simulink model "CLRC_filter_reg"  (R2024a)
settings: Solver=ode1  StartTime=0.0  StopTime=25  FixedStep=Ts  MaxStep=0.005  RelTol=1e-5
model workspace (MAT data in the model file):
  SL_ROS_VariableLengthArrays_MaxSizes.CommonInfo.ArrayTruncateAction = 'EmitWarning'
  SL_ROS_VariableLengthArrays_MaxSizes.MsgTypeMap = containers.Map
  SL_ROS_VariableLengthArrays_MaxSizes.MsgTypeMap.serialization.keys = {'gazebo_msgs/ApplyJointEffortRequest', 'sensor_msgs/JointState'}
  SL_ROS_VariableLengthArrays_MaxSizes.MsgTypeMap.serialization.values{1}.PropertyName = 'JointName'
  SL_ROS_VariableLengthArrays_MaxSizes.MsgTypeMap.serialization.values{1}.DataType = 'uint8'
  SL_ROS_VariableLengthArrays_MaxSizes.MsgTypeMap.serialization.values{1}.MaxLength = 12
  SL_ROS_VariableLengthArrays_MaxSizes.MsgTypeMap.serialization.values{2}(1).PropertyName = 'Effort'
  SL_ROS_VariableLengthArrays_MaxSizes.MsgTypeMap.serialization.values{2}(1).DataType = 'double'
  SL_ROS_VariableLengthArrays_MaxSizes.MsgTypeMap.serialization.values{2}(1).MaxLength = 128
  SL_ROS_VariableLengthArrays_MaxSizes.MsgTypeMap.serialization.values{2}(2).PropertyName = 'Name'
  SL_ROS_VariableLengthArrays_MaxSizes.MsgTypeMap.serialization.values{2}(2).DataType = 'std_msgs/String'
  SL_ROS_VariableLengthArrays_MaxSizes.MsgTypeMap.serialization.values{2}(2).MaxLength = 16
  SL_ROS_VariableLengthArrays_MaxSizes.MsgTypeMap.serialization.values{2}(3).PropertyName = 'Position'
  SL_ROS_VariableLengthArrays_MaxSizes.MsgTypeMap.serialization.values{2}(3).DataType = 'double'
  SL_ROS_VariableLengthArrays_MaxSizes.MsgTypeMap.serialization.values{2}(3).MaxLength = 7
  SL_ROS_VariableLengthArrays_MaxSizes.MsgTypeMap.serialization.values{2}(4).PropertyName = 'Velocity'
  SL_ROS_VariableLengthArrays_MaxSizes.MsgTypeMap.serialization.values{2}(4).DataType = 'double'
  SL_ROS_VariableLengthArrays_MaxSizes.MsgTypeMap.serialization.values{2}(4).MaxLength = 7
  SL_ROS_VariableLengthArrays_MaxSizes.MsgTypeMap.serialization.uniformity = 0
  SL_ROS_VariableLengthArrays_MaxSizes.MsgTypeMap.serialization.keyType = 'char'
  SL_ROS_VariableLengthArrays_MaxSizes.MsgTypeMap.serialization.valueType = 'any'
values from neighbouring files (symbols this model uses):
  alpha = 15    [Panda_run.m]
  alpha2 = 10    [Panda_run.m]
  dyn_par = opt_par()    [Panda_run.m]
  fricpar = FrictionPar()    [Panda_run.m]
  GammaW = 0.4*eye(N)    [Panda_run.m]
  invP = inv(P*P')*P    [Panda_run.m]
  kapa1 = 1    [Panda_run.m]
  kapa2 = 0    [Panda_run.m]
  Kc = diag([10,10,10,10,4,4,2.5])    [Panda_run.m]
  Lambda = 3*eye(7)    [Panda_run.m]
  P0 = 0.04    [Panda_run.m]
  P1 = 1    [Panda_run.m]
  q0 = [0, -0.60, 0, -2.25, 0, 1.5, 0.8]'    [Panda_run.m]
  robot_par = [basepar;fricpar]    [Panda_run.m]
  SD = 0.0    (= 0)    [Panda_run.m]
  taud = 25    [Panda_run.m]
  Ts = 0.0005    [Panda_run.m]
  vari = SD^2    [DDF_Test_main.m]    (also in Panda_run.m = 0; RegComp_main.m)
libraries: matrix_library x3
settings Model: SimulationMode=accelerator  Creator=STT  LastModifiedBy=SYSU-RCLLab-G
settings OptimizationCC: DefaultParameterBehavior=Inlined  EnhancedBackFolding=on  PassReuseOutputArgsAs=Individual arguments  ZeroExternalMemoryAtStartup=off  ZeroInternalMemoryAtStartup=off  MaxStackSize=64  AccelVerboseBuild=on  OptimizeBlockOrder=speed  DifferentSizesBufferReuse=on  OptimizationCustomize=off  EfficientTunableParamExpr=on
settings DebuggingCC: ArtificialAlgebraicLoopMsg=error  ParameterTunabilityLossMsg=error  UnconnectedInputMsg=warning  UnconnectedOutputMsg=warning  UnconnectedLineMsg=warning
settings ModelReferenceCC: EnableRefExpFcnMdlSchedulingChecks=on
settings SFSimCC: MATLABDynamicMemAlloc=off
settings RTWCC: Description=Embedded Coder  SystemTargetFile=ert.tlc  TemplateMakefile=ert_default_tmf  Toolchain=Catkin  GPUComputeCapability=3.5  DLArmComputeVersion=19.05
settings CodeAppCC: ForceParamTrailComments=on  IgnoreCustomStorageClasses=off  OperatorAnnotations=on  SimulinkDataObjDesc=on  SFDataObjDesc=on  InsertBlockDesc=on
settings ERTTargetCC: SupportContinuousTime=on  SupportVariableSizeSignals=on  ExtMode=on  ExtModeMexArgs='192.168.175.128' 0 17725  ERTCustomFileTemplate=example_file_process.tlc

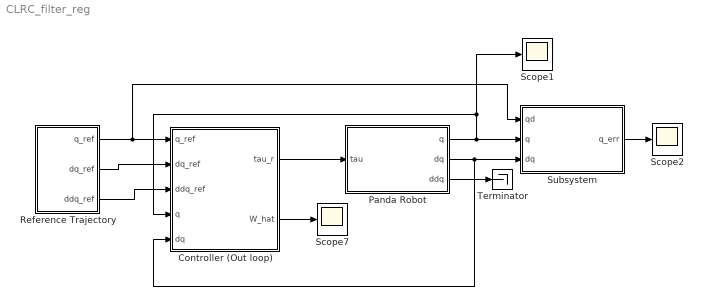
== system CLRC_filter_reg ==
  Controller (Out loop) : Subsystem  SystemSampleTime=1e-3
  Panda Robot : Subsystem
  Reference Trajectory : Subsystem
  Scope1 : Scope
  Scope2 : Scope
  Scope7 : Scope
  Subsystem : Subsystem
  Terminator : Terminator
  wires:
  Controller (Out loop)/2(W_hat) -> Scope7/1
  Controller (Out loop)/1(tau_r) -> Panda Robot/1(tau)
  Reference Trajectory/1(q_ref) -> Subsystem/1(qd), Controller (Out loop)/1(q_ref)
  Reference Trajectory/2(dq_ref) -> Controller (Out loop)/2(dq_ref)
  Reference Trajectory/3(ddq_ref) -> Controller (Out loop)/3(ddq_ref)
  Panda Robot/2(dq) -> Subsystem/3(dq), Controller (Out loop)/5(dq)
  Subsystem/1(q_err) -> Scope2/1
  Panda Robot/1(q) -> Scope1/1, Controller (Out loop)/4(q), Subsystem/2(q)
  Panda Robot/3(ddq) -> Terminator/1

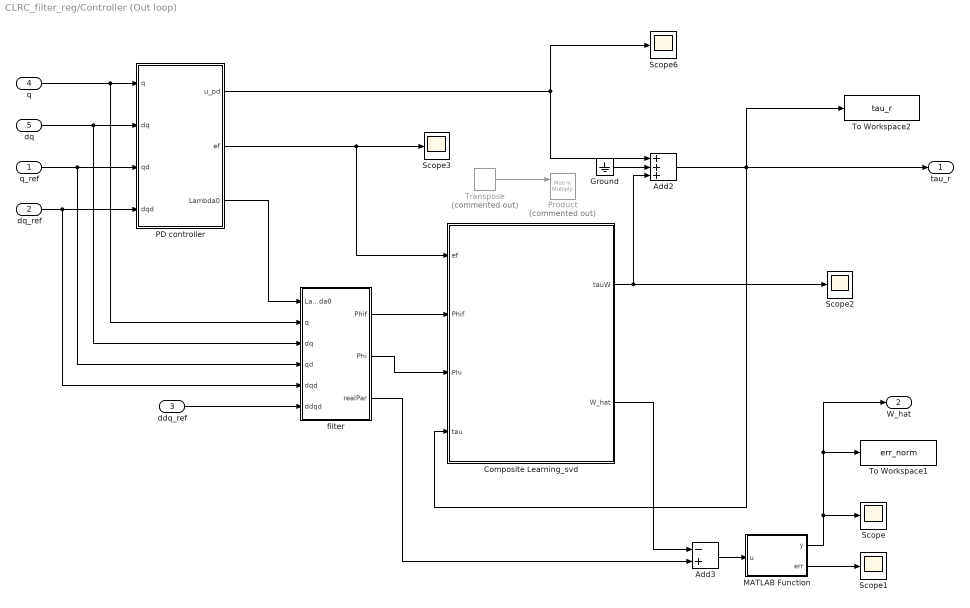
== system CLRC_filter_reg/Controller (Out loop) ==
  q_ref : Inport
  dq_ref : Inport  Port=2
  ddq_ref : Inport  Port=3
  q : Inport  Port=4
  dq : Inport  Port=5
  Add2 : Sum  Inputs=+++
  Add3 : Sum  Inputs=-+
  Composite Learning_svd : Subsystem
  Ground : Ground
  MATLAB Function : MATLAB Function  TreatAsAtomicUnit=on
  PD controller : Subsystem
  Product : Product  Commented=on  Multiplication=Matrix(*)
  Scope{,1..3,6} (5 alike) : Scope
  To Workspace1 : ToWorkspace  VariableName=err_norm  SaveFormat=Timeseries  SampleTime=-1
  To Workspace2 : ToWorkspace  VariableName=tau_r  SaveFormat=Timeseries  SampleTime=-1
  Transpose : matrix_library/Transpose  Commented=on
  filter : Subsystem
  tau_r : Outport
  W_hat : Outport  Port=2
  wires:
  q_ref/1 -> filter/4(qd), PD controller/3(qd)
  dq_ref/1 -> filter/5(dqd), PD controller/4(dqd)
  dq/1 -> filter/3(dq), PD controller/2(dq)
  ddq_ref/1 -> filter/6(ddqd)
  Add3/1 -> MATLAB Function/1(u)
  MATLAB Function/1(y) -> W_hat/1, To Workspace1/1, Scope/1
  filter/1(Phif) -> Composite Learning_svd/2(Phif)
  filter/2(Phi) -> Composite Learning_svd/3(Phi)
  MATLAB Function/2(err) -> Scope1/1
  filter/3(realPar) -> Add3/2
  Transpose/1 -> Product/1
  Composite Learning_svd/1(tauW) -> Add2/3, Scope2/1
  q/1 -> filter/2(q), PD controller/1(q)
  Composite Learning_svd/2(W_hat) -> Add3/1
  Add2/1 -> Composite Learning_svd/4(tau), tau_r/1, To Workspace2/1
  PD controller/3(Lambda0) -> filter/1(Lambda0)
  PD controller/2(ef) -> Scope3/1, Composite Learning_svd/1(ef)
  PD controller/1(u_pd) -> Add2/1, Scope6/1
  Ground/1 -> Add2/2

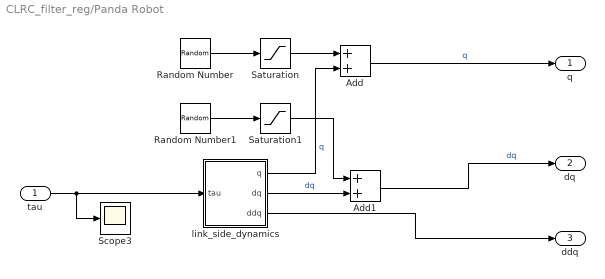
== system CLRC_filter_reg/Panda Robot ==
  tau : Inport
  Add : Sum
  Add1 : Sum
  Random Number : RandomNumber  Variance=vari  SampleTime=Ts
  Random Number1 : RandomNumber  Variance=vari  SampleTime=Ts
  Saturation : Saturate  UpperLimit=3*SD  LowerLimit=-3*SD
  Saturation1 : Saturate  UpperLimit=3*SD  LowerLimit=-3*SD
  Scope3 : Scope
  link_side_dynamics : Subsystem
  q : Outport
  dq : Outport  Port=2
  ddq : Outport  Port=3
  wires:
  link_side_dynamics/1(q) -> Add/2  "q"
  tau/1 -> link_side_dynamics/1(tau), Scope3/1
  Random Number/1 -> Saturation/1
  Saturation/1 -> Add/1
  Random Number1/1 -> Saturation1/1
  link_side_dynamics/2(dq) -> Add1/2  "dq"
  Add/1 -> q/1  "q"
  Add1/1 -> dq/1  "dq"
  Saturation1/1 -> Add1/1
  link_side_dynamics/3(ddq) -> ddq/1

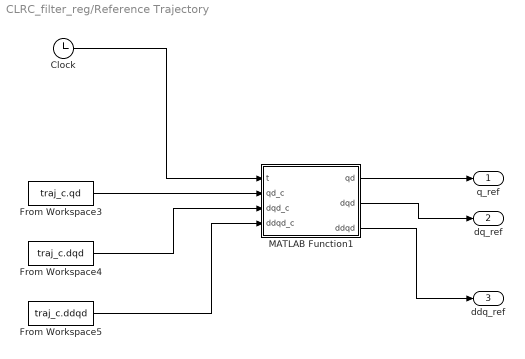
== system CLRC_filter_reg/Reference Trajectory ==
  Clock : Clock
  From Workspace3 : FromWorkspace  VariableName=traj_c.qd
  From Workspace4 : FromWorkspace  VariableName=traj_c.dqd
  From Workspace5 : FromWorkspace  VariableName=traj_c.ddqd
  MATLAB Function1 : MATLAB Function  TreatAsAtomicUnit=on
  q_ref : Outport
  dq_ref : Outport  Port=2
  ddq_ref : Outport  Port=3
  wires:
  Clock/1 -> MATLAB Function1/1(t)
  MATLAB Function1/1(qd) -> q_ref/1
  MATLAB Function1/2(dqd) -> dq_ref/1
  MATLAB Function1/3(ddqd) -> ddq_ref/1
  From Workspace3/1 -> MATLAB Function1/2(qd_c)
  From Workspace4/1 -> MATLAB Function1/3(dqd_c)
  From Workspace5/1 -> MATLAB Function1/4(ddqd_c)

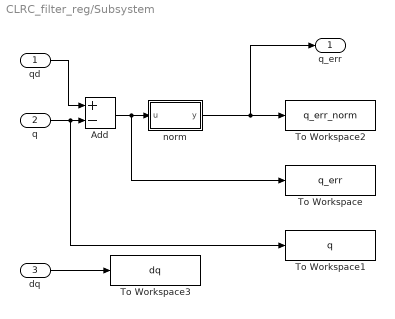
== system CLRC_filter_reg/Subsystem ==
  qd : Inport
  q : Inport  Port=2
  dq : Inport  Port=3
  Add : Sum  Inputs=+-
  To Workspace : ToWorkspace  VariableName=q_err  SaveFormat=Timeseries  SampleTime=-1
  To Workspace1 : ToWorkspace  VariableName=q  SaveFormat=Timeseries  SampleTime=-1
  To Workspace2 : ToWorkspace  VariableName=q_err_norm  SaveFormat=Timeseries  SampleTime=-1
  To Workspace3 : ToWorkspace  VariableName=dq  SaveFormat=Timeseries  SampleTime=-1
  norm : MATLAB Function  TreatAsAtomicUnit=on
  q_err : Outport
  wires:
  norm/1(y) -> q_err/1, To Workspace2/1
  q/1 -> To Workspace1/1, Add/2
  qd/1 -> Add/1
  Add/1 -> norm/1(u), To Workspace/1
  dq/1 -> To Workspace3/1

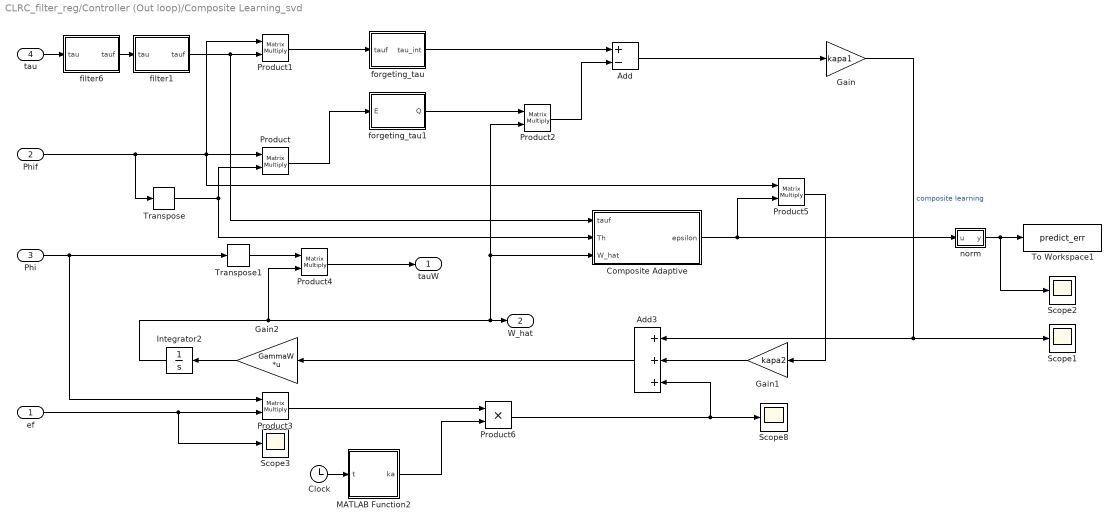
== system CLRC_filter_reg/Controller (Out loop)/Composite Learning_svd ==
  ef : Inport
  Phif : Inport  Port=2
  Phi : Inport  Port=3
  tau : Inport  Port=4
  Add : Sum  Inputs=+-
  Add3 : Sum  Inputs=+++
  Clock : Clock
  Composite Adaptive : Subsystem
  Gain : Gain  Gain=kapa1
  Gain1 : Gain  Gain=kapa2
  Gain2 : Gain  Gain=GammaW  Multiplication=Matrix(K*u)
  Integrator2 : Integrator  UpperSaturationLimit=10  LowerSaturationLimit=-1
  MATLAB Function2 : MATLAB Function  TreatAsAtomicUnit=on
  Product{,1..5} (6 alike) : Product  Multiplication=Matrix(*)
  Product6 : Product
  Scope{1..3,8} (4 alike) : Scope
  To Workspace1 : ToWorkspace  VariableName=predict_err  SaveFormat=Timeseries  SampleTime=-1
  Transpose : matrix_library/Transpose
  Transpose1 : matrix_library/Transpose
  filter1 : Subsystem
  filter6 : Subsystem
  forgeting_tau : Subsystem
  forgeting_tau1 : Subsystem
  norm : MATLAB Function  TreatAsAtomicUnit=on
  tauW : Outport
  W_hat : Outport  Port=2
  wires:
  Transpose/1 -> Composite Adaptive/2(Th), Product/2
  ef/1 -> Scope3/1, Product3/2
  Phi/1 -> Transpose1/1, Product3/1
  Transpose1/1 -> Product4/1
  Phif/1 -> Product1/1, Product5/1, Product/1, Transpose/1
  Gain2/1 -> Integrator2/1
  Add3/1 -> Gain2/1
  Composite Adaptive/1(epsilon) -> Product5/2, norm/1(u)
  Product4/1 -> tauW/1
  norm/1(y) -> Scope2/1, To Workspace1/1
  tau/1 -> filter6/1(tau)
  filter1/1(tauf) -> Composite Adaptive/1(tauf), Product1/2
  Product3/1 -> Product6/1
  Gain/1 -> Add3/1, Scope1/1  "composite learning"
  Integrator2/1 -> Product4/2, Product2/2, Composite Adaptive/3(W_hat), W_hat/1
  Product/1 -> forgeting_tau1/1(E)
  Product1/1 -> forgeting_tau/1(tauf)
  forgeting_tau1/1(Q) -> Product2/1
  forgeting_tau/1(tau_int) -> Add/1
  Product2/1 -> Add/2
  Add/1 -> Gain/1
  filter6/1(tauf) -> filter1/1(tau)
  Clock/1 -> MATLAB Function2/1(t)
  MATLAB Function2/1(ka) -> Product6/2
  Product5/1 -> Gain1/1
  Product6/1 -> Add3/3, Scope8/1
  Gain1/1 -> Add3/2

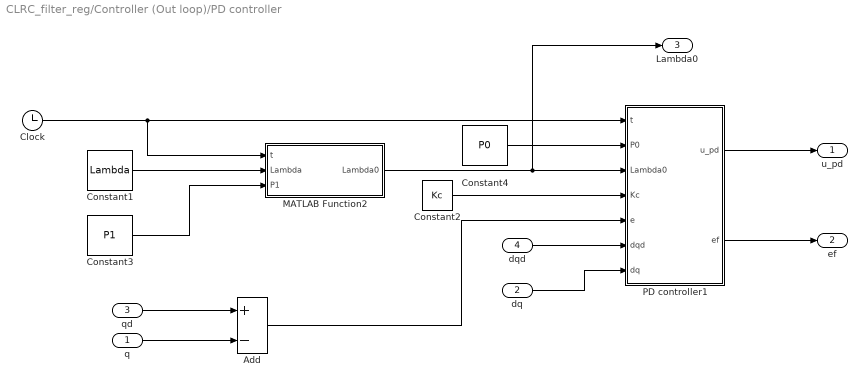
== system CLRC_filter_reg/Controller (Out loop)/PD controller ==
  q : Inport
  dq : Inport  Port=2
  qd : Inport  Port=3
  dqd : Inport  Port=4
  Add : Sum  Inputs=+-
  Clock : Clock
  Constant1 : Constant  Value=Lambda
  Constant2 : Constant  Value=Kc
  Constant3 : Constant  Value=P1
  Constant4 : Constant  Value=P0
  MATLAB Function2 : MATLAB Function  TreatAsAtomicUnit=on
  PD controller1 : MATLAB Function  TreatAsAtomicUnit=on
  u_pd : Outport
  ef : Outport  Port=2
  Lambda0 : Outport  Port=3
  wires:
  PD controller1/1(u_pd) -> u_pd/1
  Constant4/1 -> PD controller1/2(P0)
  Clock/1 -> MATLAB Function2/1(t), PD controller1/1(t)
  Add/1 -> PD controller1/5(e)
  MATLAB Function2/1(Lambda0) -> Lambda0/1, PD controller1/3(Lambda0)
  Constant1/1 -> MATLAB Function2/2(Lambda)
  Constant3/1 -> MATLAB Function2/3(P1)
  Constant2/1 -> PD controller1/4(Kc)
  PD controller1/2(ef) -> ef/1
  q/1 -> Add/2
  qd/1 -> Add/1
  dq/1 -> PD controller1/7(dq)
  dqd/1 -> PD controller1/6(dqd)

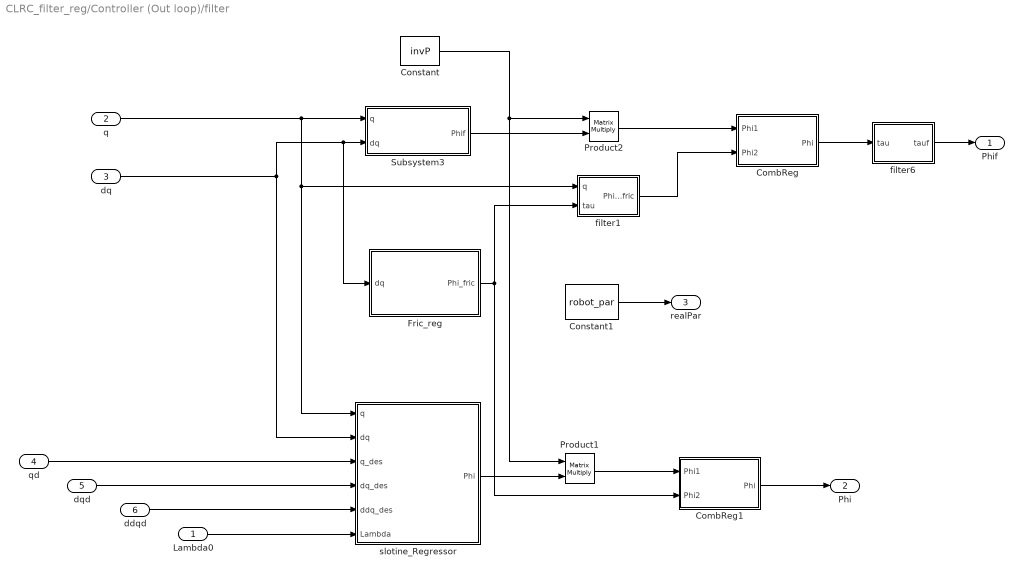
== system CLRC_filter_reg/Controller (Out loop)/filter ==
  Lambda0 : Inport
  q : Inport  Port=2
  dq : Inport  Port=3
  qd : Inport  Port=4
  dqd : Inport  Port=5
  ddqd : Inport  Port=6
  CombReg : MATLAB Function  TreatAsAtomicUnit=on
  CombReg1 : MATLAB Function  TreatAsAtomicUnit=on
  Constant : Constant  Value=invP
  Constant1 : Constant  Value=robot_par
  Fric_reg : MATLAB Function  TreatAsAtomicUnit=on
  Product1 : Product  Multiplication=Matrix(*)
  Product2 : Product  Multiplication=Matrix(*)
  Subsystem3 : Subsystem
  filter1 : Subsystem
  filter6 : Subsystem
  slotine_Regressor : MATLAB Function  TreatAsAtomicUnit=on
  Phif : Outport
  Phi : Outport  Port=2
  realPar : Outport  Port=3
  wires:
  qd/1 -> slotine_Regressor/3(q_des)
  dqd/1 -> slotine_Regressor/4(dq_des)
  ddqd/1 -> slotine_Regressor/5(ddq_des)
  Lambda0/1 -> slotine_Regressor/6(Lambda)
  q/1 -> filter1/1(q), slotine_Regressor/1(q), Subsystem3/1(q)
  dq/1 -> Fric_reg/1(dq), Subsystem3/2(dq), slotine_Regressor/2(dq)
  Constant1/1 -> realPar/1
  filter6/1(tauf) -> Phif/1
  Fric_reg/1(Phi_fric) -> filter1/2(tau), CombReg1/2(Phi2)
  filter1/1(Phif_fric) -> CombReg/2(Phi2)
  slotine_Regressor/1(Phi) -> Product1/2
  CombReg/1(Phi) -> filter6/1(tau)
  CombReg1/1(Phi) -> Phi/1
  Constant/1 -> Product2/1, Product1/1
  Product1/1 -> CombReg1/1(Phi1)
  Product2/1 -> CombReg/1(Phi1)
  Subsystem3/1(Phif) -> Product2/2

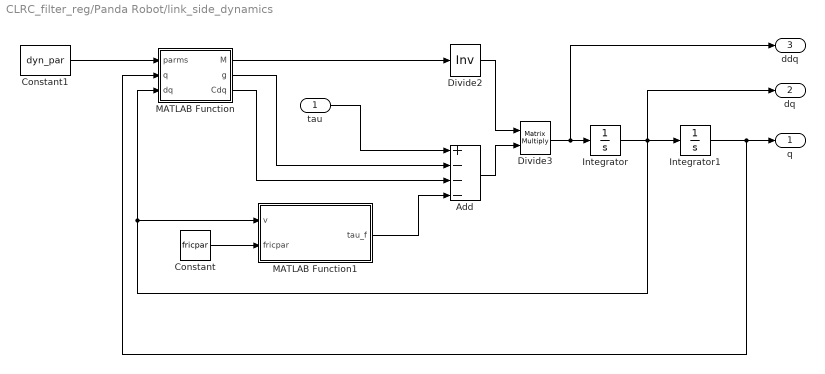
== system CLRC_filter_reg/Panda Robot/link_side_dynamics ==
  tau : Inport
  Add : Sum  Inputs=+---
  Constant : Constant  Value=fricpar
  Constant1 : Constant  Value=dyn_par
  Divide2 : Product  Inputs=/  Multiplication=Matrix(*)
  Divide3 : Product  Inputs=**  Multiplication=Matrix(*)
  Integrator : Integrator  InitialCondition=zeros(7,1)
  Integrator1 : Integrator  InitialCondition=q0
  MATLAB Function : MATLAB Function  TreatAsAtomicUnit=on
  MATLAB Function1 : MATLAB Function  TreatAsAtomicUnit=on
  q : Outport
  dq : Outport  Port=2
  ddq : Outport  Port=3
  wires:
  Divide3/1 -> Integrator/1, ddq/1
  tau/1 -> Add/1
  Integrator1/1 -> q/1, MATLAB Function/2(q)
  Constant/1 -> MATLAB Function1/2(fricpar)
  Add/1 -> Divide3/2
  Divide2/1 -> Divide3/1
  MATLAB Function1/1(tau_f) -> Add/4
  Integrator/1 -> MATLAB Function/3(dq), MATLAB Function1/1(v), Integrator1/1, dq/1
  MATLAB Function/1(M) -> Divide2/1
  MATLAB Function/3(Cdq) -> Add/3
  Constant1/1 -> MATLAB Function/1(parms)
  MATLAB Function/2(g) -> Add/2

== system CLRC_filter_reg/Controller (Out loop)/Composite Learning_svd/Composite Adaptive ==
  tauf : Inport
  Th : Inport  Port=2
  W_hat : Inport  Port=3
  Add1 : Sum  Inputs=+-
  Product6 : Product  Multiplication=Matrix(*)
  epsilon : Outport
  wires:
  Add1/1 -> epsilon/1
  Product6/1 -> Add1/2
  tauf/1 -> Add1/1
  Th/1 -> Product6/1
  W_hat/1 -> Product6/2

== system CLRC_filter_reg/Controller (Out loop)/Composite Learning_svd/filter1 ==
  tau : Inport
  Add : Sum  Inputs=+-
  Gain : Gain  Gain=alpha2
  Integrator : Integrator  UpperSaturationLimit=20  LowerSaturationLimit=-20
  tauf : Outport
  wires:
  tau/1 -> Add/1
  Add/1 -> Gain/1
  Gain/1 -> Integrator/1
  Integrator/1 -> Add/2, tauf/1

== system CLRC_filter_reg/Controller (Out loop)/Composite Learning_svd/filter6 ==
  tau : Inport
  Add : Sum  Inputs=+-
  Gain : Gain  Gain=alpha
  Integrator : Integrator  UpperSaturationLimit=20  LowerSaturationLimit=-20
  tauf : Outport
  wires:
  tau/1 -> Add/1
  Add/1 -> Gain/1
  Gain/1 -> Integrator/1
  Integrator/1 -> Add/2, tauf/1

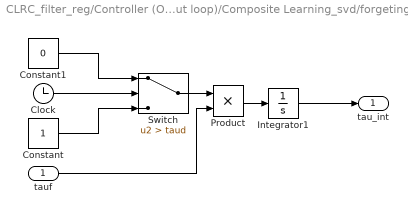
== system CLRC_filter_reg/Controller (Out loop)/Composite Learning_svd/forgeting_tau ==
  tauf : Inport
  Clock : Clock
  Constant : Constant
  Constant1 : Constant  Value=0
  Integrator1 : Integrator  UpperSaturationLimit=20  LowerSaturationLimit=-20
  Product : Product
  Switch : Switch  Criteria=u2 > Threshold  Threshold=taud  SaturateOnIntegerOverflow=off  InputSameDT=off
  tau_int : Outport
  wires:
  tauf/1 -> Product/2
  Clock/1 -> Switch/2
  Integrator1/1 -> tau_int/1
  Constant/1 -> Switch/3
  Constant1/1 -> Switch/1
  Switch/1 -> Product/1
  Product/1 -> Integrator1/1

== system CLRC_filter_reg/Controller (Out loop)/Composite Learning_svd/forgeting_tau1 ==
  E : Inport
  Clock : Clock
  Constant : Constant
  Constant1 : Constant  Value=0
  Integrator1 : Integrator  UpperSaturationLimit=20  LowerSaturationLimit=-20
  Product : Product
  Switch : Switch  Criteria=u2 > Threshold  Threshold=taud  SaturateOnIntegerOverflow=off  InputSameDT=off
  Q : Outport
  wires:
  E/1 -> Product/2
  Clock/1 -> Switch/2
  Integrator1/1 -> Q/1
  Constant/1 -> Switch/3
  Constant1/1 -> Switch/1
  Switch/1 -> Product/1
  Product/1 -> Integrator1/1

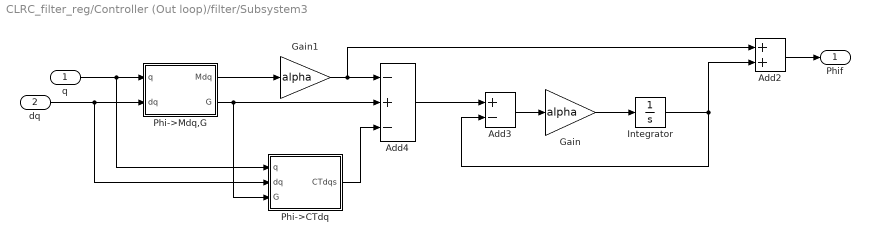
== system CLRC_filter_reg/Controller (Out loop)/filter/Subsystem3 ==
  q : Inport
  dq : Inport  Port=2
  Add2 : Sum
  Add3 : Sum  Inputs=+-
  Add4 : Sum  Inputs=-+-
  Gain : Gain  Gain=alpha
  Gain1 : Gain  Gain=alpha
  Integrator : Integrator  UpperSaturationLimit=20  LowerSaturationLimit=-20
  Phi->CTdq : MATLAB Function  TreatAsAtomicUnit=on
  Phi->Mdq,G : MATLAB Function  TreatAsAtomicUnit=on
  Phif : Outport
  wires:
  Add4/1 -> Add3/1
  Add2/1 -> Phif/1
  Add3/1 -> Gain/1
  Gain/1 -> Integrator/1
  q/1 -> Phi->CTdq/1(q), Phi->Mdq,G/1(q)
  dq/1 -> Phi->CTdq/2(dq), Phi->Mdq,G/2(dq)
  Phi->Mdq,G/1(Mdq) -> Gain1/1
  Gain1/1 -> Add2/1, Add4/1
  Integrator/1 -> Add2/2, Add3/2
  Phi->CTdq/1(CTdqs) -> Add4/3
  Phi->Mdq,G/2(G) -> Add4/2, Phi->CTdq/3(G)

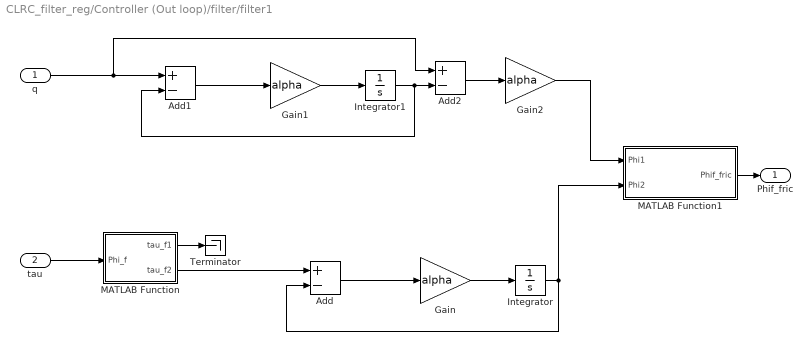
== system CLRC_filter_reg/Controller (Out loop)/filter/filter1 ==
  q : Inport
  tau : Inport  Port=2
  Add : Sum  Inputs=+-
  Add1 : Sum  Inputs=+-
  Add2 : Sum  Inputs=+-
  Gain : Gain  Gain=alpha
  Gain1 : Gain  Gain=alpha
  Gain2 : Gain  Gain=alpha
  Integrator : Integrator  UpperSaturationLimit=20  LowerSaturationLimit=-20
  Integrator1 : Integrator  InitialCondition=q0  UpperSaturationLimit=20  LowerSaturationLimit=-20
  MATLAB Function : MATLAB Function  TreatAsAtomicUnit=on
  MATLAB Function1 : MATLAB Function  TreatAsAtomicUnit=on
  Terminator : Terminator
  Phif_fric : Outport
  wires:
  Add/1 -> Gain/1
  Gain/1 -> Integrator/1
  Integrator/1 -> MATLAB Function1/2(Phi2), Add/2
  tau/1 -> MATLAB Function/1(Phi_f)
  MATLAB Function/2(tau_f2) -> Add/1
  Integrator1/1 -> Add1/2, Add2/2
  Gain1/1 -> Integrator1/1
  Add1/1 -> Gain1/1
  q/1 -> Add1/1, Add2/1
  Add2/1 -> Gain2/1
  MATLAB Function1/1(Phif_fric) -> Phif_fric/1
  Gain2/1 -> MATLAB Function1/1(Phi1)
  MATLAB Function/1(tau_f1) -> Terminator/1

== system CLRC_filter_reg/Controller (Out loop)/filter/filter6 ==
  tau : Inport
  Add : Sum  Inputs=+-
  Gain : Gain  Gain=alpha2
  Integrator : Integrator  UpperSaturationLimit=20  LowerSaturationLimit=-20
  tauf : Outport
  wires:
  tau/1 -> Add/1
  Add/1 -> Gain/1
  Gain/1 -> Integrator/1
  Integrator/1 -> Add/2, tauf/1

== matlab function CLRC_filter_reg/Controller (Out loop)/filter/CombReg1 ==
  data: Phi1 input; Phi output; Phi2 input
function Phi = fcn(Phi1,Phi2)

Phi = [Phi1;Phi2];

== matlab function CLRC_filter_reg/Controller (Out loop)/filter/filter1/MATLAB Function ==
  data: Phi_f input; tau_f1 output; tau_f2 output
function [tau_f1,tau_f2] = fcn(Phi_f)
tau_f1=Phi_f(1:7,:);
tau_f2 = Phi_f(8:end,:);

== matlab function CLRC_filter_reg/Controller (Out loop)/filter/filter1/MATLAB Function1 ==
  data: Phi1 input; Phif_fric output; Phi2 input
function Phif_fric = fcn(Phi1,Phi2)
Phif_fric=[diag(Phi1);Phi2];

== matlab function CLRC_filter_reg/Controller (Out loop)/Composite Learning_svd/MATLAB Function2 ==
  data: t input; ka output
function ka= fcn(t)


if t<40
    ka=1;
elseif t<100
    ka=1-0.5*(1+tanh((t-70)/5));
else
    ka=0;
end

== matlab function CLRC_filter_reg/Controller (Out loop)/PD controller/PD controller1 ==
  data: t input; P0 input; Lambda0 input; Kc input; e input; dqd input; u_pd output; dq input; ef output
function [u_pd,ef]= fcn(t,P0,Lambda0,Kc,e,dqd,dq)


%% Kc
% P0=0.02;
if t<40
    Kc0=Kc;
elseif t<100
    Kc0=Kc-0.5*(1+tanh((t-70)/5))*(1-P0)*Kc;
else
    Kc0=P0*Kc;
end
dqr=(dqd+Lambda0*e);

ef=dqr-dq;

u_pd = Kc0*ef;

== matlab function CLRC_filter_reg/Panda Robot/link_side_dynamics/MATLAB Function ==
  data: parms input; M output; q input; dq input; g output; Cdq output
function [M,g,Cdq] = fcn(parms,q,dq)

M= Mass(parms,q);

g=gravity(parms,q);

Cdq= CoriolisVector(parms,q,dq);

== matlab function CLRC_filter_reg/Controller (Out loop)/MATLAB Function ==
  data: u input; y output; err output
function [y,err]= fcn(u)

y = norm(u);
err=abs(u);

== matlab function CLRC_filter_reg/Controller (Out loop)/PD controller/MATLAB Function2 ==
  data: t input; Lambda0 output; Lambda input; P1 input
function Lambda0= fcn(t,Lambda,P1)


if t<40
    Lambda0=Lambda;
elseif t<100
    Lambda0=Lambda-0.5*(1+tanh((t-70)/5))*(1-P1)*Lambda;
else
    Lambda0=P1*Lambda;
end

== matlab function CLRC_filter_reg/Controller (Out loop)/filter/Subsystem3/Phi->Mdq,G ==
  data: q input; Mdq output; dq input; G output
function [Mdq,G] = fcn(q,dq)


vec0=zeros(7,1);


% G=Base_Regressor_Panda_43(q,vec0,vec0);
% Mdq=Base_Regressor_Panda_43(q,vec0,dq)-G;
G=Regressor_Panda_full(q,vec0,vec0);

Mdq=Regressor_Panda_full(q,vec0,dq)-G;

== matlab function CLRC_filter_reg/Subsystem/norm ==
  data: u input; y output
function y = fcn(u)

y = norm(u);

== matlab function CLRC_filter_reg/Panda Robot/link_side_dynamics/MATLAB Function1 ==
  data: v input; tau_f output; fricpar input
function tau_f = signFriction(v,fricpar)
 % f_v =[0.0665, 0.1987, 0.0399, 0.2257,  0.1023, -0.0132, 0.0638]';
 % f_c =[0.245, 0.1523, 0.1827, 0.3591, 0.2669, 0.1658, 0.2109 ]';
 % f_o =[-0.1073,-0.1566,-0.0686,-0.2522,0.0045,0.0910,-0.0127]';
 % tau_f = f_v.*v+f_c.*tanh(300*v)+f_o;


 tau_f = Regressor_fric(v)'*fricpar;

== matlab function CLRC_filter_reg/Controller (Out loop)/filter/Fric_reg ==
  data: dq input; Phi_fric output
function Phi_fric = fcn(dq)

Phi_fric = Regressor_fric(dq);

== matlab function CLRC_filter_reg/Controller (Out loop)/filter/slotine_Regressor ==
  data: q input; Phi output; dq input; q_des input; dq_des input; ddq_des input; Lambda input
function Phi = fcn(q,dq,q_des,dq_des,ddq_des,Lambda)
e1=q-q_des;
de1=dq-dq_des;


dqr=(dq_des-Lambda*e1);

ddqr=ddq_des-Lambda*de1;

Phi=Base_Slotine_Panda(q,dq,dqr,ddqr);

== matlab function CLRC_filter_reg/Controller (Out loop)/filter/Subsystem3/Phi->CTdq ==
  data: q input; CTdqs output; dq input; G input
function CTdqs = fcn(q,dq,G)

CTdqs=Coriolis_Reg(q,dq,G);
% I=eye(7);
% CTdqs=zeros(7,64)';
% for k=1:7
%     CorReg=Coriolis_Reg(q,dq,I(:,k));
%     for i=1:7
%         CTdq(k,:)=CTdq(k,:)+dq(i)*CorReg(i,:);
%     end
% end
% CTdqs=CTdq';


% CTdqs=[Coriolis_Reg(q,dq,I(:,1))'*dq,Coriolis_Reg(q,dq,I(:,2))'*dq,Coriolis_Reg(q,dq,I(:,3))'*dq,...
%     Coriolis_Reg(q,dq,I(:,4))'*dq,Coriolis_Reg(q,dq,I(:,5))'*dq,Coriolis_Reg(q,dq,I(:,6))'*dq,...
%     Coriolis_Reg(q,dq,I(:,7))'*dq];

== matlab function CLRC_filter_reg/Reference Trajectory/MATLAB Function1 ==
  data: t input; qd output; dqd output; ddqd output; qd_c input; dqd_c input; ddqd_c input
function [qd,dqd,ddqd] = fcn(t,qd_c,dqd_c,ddqd_c)

if t<=100
    T=[0,3,6,9,13,17,20,23];
    P=[0, -0.60, 0, -2.25, 0, 1.5, 0.8;
        -0.75, 0.25, 0, -0.8, -1.2, 0.5, -1.8;
        1.5, 0.6, -0.83, -0.5, 1.04, 1.6, -2.0;
        0.25, -0.55, 0.3, -1.75, 0.25, 0.75, 0.50;
        -1.20, 0.84, -0.85, -1.0, 1.07, 2.55, 2.05;
        -2.25, -1.2, 2.23, -0.63, -0.54, 2.8, 1.3;
        -0.25, 1.0, -0.23, -1.33, -0.24, 1.1, -2.5;
        0, -0.60, 0, -2.25, 0, 1.5, 0.8];
    [qd,dqd,ddqd]=traj_gen_fun(t,T,P);
% elseif t<=120
%     T=[100,105];
%     P=[0, -0.60, 0, -2.25, 0, 1.5, 0.8;
%        0, 0, 0, -pi/2, 0, pi, pi/4];
%     [qd,dqd,ddqd]=traj_gen_fun(t,T,P);
elseif t<=150
    qd=qd_c;dqd=dqd_c;ddqd=ddqd_c;
else
    qd=[0, -0.60, 0, -2.25, 0, 1.5, 0.8]';
    dqd=zeros(7,1);
    ddqd=zeros(7,1);
    % T=[160,165];
    % P=[0, 0, 0, -pi/2, 0, pi, pi/4;
    %    0, -0.60, 0, -2.25, 0, 1.5, 0.8];
    % [qd,dqd,ddqd]=traj_gen_fun(t,T,P);
end

== matlab function CLRC_filter_reg/Controller (Out loop)/Composite Learning_svd/norm ==
  data: u input; y output
function y= fcn(u)

y = norm(u);

== matlab function CLRC_filter_reg/Controller (Out loop)/filter/CombReg ==
  data: Phi1 input; Phi output; Phi2 input
function Phi = fcn(Phi1,Phi2)

Phi = [Phi1;Phi2];
